simulink library "readers"  (R2020a)
settings: Solver=VariableStepAuto  StartTime=0.0  StopTime=10.0  RelTol=1e-3
settings Model: Creator=thomas  LastModifiedBy=thomas

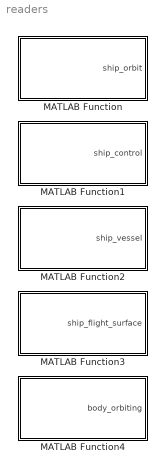
== system readers ==
  MATLAB Function : MATLAB Function  TreatAsAtomicUnit=on
  MATLAB Function1 : MATLAB Function  TreatAsAtomicUnit=on
  MATLAB Function2 : MATLAB Function  TreatAsAtomicUnit=on
  MATLAB Function3 : MATLAB Function  TreatAsAtomicUnit=on
  MATLAB Function4 : MATLAB Function  TreatAsAtomicUnit=on

== matlab function readers/MATLAB Function1 ==
  data: ship_control output Bus: ShipControl
function ship_control = read_control
    coder.extrinsic('evalin');
    ship_control.sas = false;
    ship_control.sas = evalin('base', 'vessel_control.getSAS();');
    ship_control.rcs = false;
    ship_control.rcs = evalin('base', 'vessel_control.getRCS();');
    ship_control.reaction_wheels = false;
    ship_control.reaction_wheels = evalin('base', 'vessel_control.getReactionWheels();');
    ship_control.gear = false;
    ship_control.gear = evalin('base', 'vessel_control.getGear();');
    ship_control.legs = false;
    ship_control.legs = evalin('base', 'vessel_control.getLegs();');
    ship_control.wheels = false;
    ship_control.wheels = evalin('base', 'vessel_control.getWheels();');
    ship_control.lights = false;
    ship_control.lights = evalin('base', 'vessel_control.getLights();');
    ship_control.brakes = false;
    ship_control.brakes = evalin('base', 'vessel_control.getBrakes();');
    ship_control.antennas = false;
    ship_control.antennas = evalin('base', 'vessel_control.getAntennas();');
    ship_control.cargo_bays = false;
    ship_control.cargo_bays = evalin('base', 'vessel_control.getCargoBays();');
    ship_control.intakes = false;
    ship_control.intakes = evalin('base', 'vessel_control.getIntakes();');
    ship_control.parachutes = false;
    ship_control.parachutes = evalin('base', 'vessel_control.getParachutes();');
    ship_control.radiators = false;
    ship_control.radiators = evalin('base', 'vessel_control.getRadiators();');
    ship_control.resource_harvesters = false;
    ship_control.resource_harvesters = evalin('base', 'vessel_control.getResourceHarvesters();');
    ship_control.resource_harvesters_active = false;
    ship_control.resource_harvesters_active = evalin('base', 'vessel_control.getResourceHarvestersActive();');
    ship_control.solar_panels = false;
    ship_control.solar_panels = evalin('base', 'vessel_control.getSolarPanels();');
    ship_control.abort = false;
    ship_control.abort = evalin('base', 'vessel_control.getAbort();');
    ship_control.throttle = 0.0;
    ship_control.throttle = evalin('base', 'vessel_control.getThrottle();');
    ship_control.pitch = 0.0;
    ship_control.pitch = evalin('base', 'vessel_control.getPitch();');
    ship_control.yaw = 0.0;
    ship_control.yaw = evalin('base', 'vessel_control.getYaw();');
    ship_control.roll = 0.0;
    ship_control.roll = evalin('base', 'vessel_control.getRoll();');
    ship_control.forward = 0.0;
    ship_control.forward = evalin('base', 'vessel_control.getForward();');
    ship_control.up = 0.0;
    ship_control.up = evalin('base', 'vessel_control.getUp();');
    ship_control.right = 0.0;
    ship_control.right = evalin('base', 'vessel_control.getRight();');
    ship_control.wheel_throttle = 0.0;
    ship_control.wheel_throttle = evalin('base', 'vessel_control.getWheelThrottle();');
    ship_control.wheel_steering = 0.0;
    ship_control.wheel_steering = evalin('base', 'vessel_control.getWheelSteering();');
    ship_control.current_stage = uint8(0);
    ship_control.current_stage = evalin('base', 'uint8(vessel_control.getCurrentStage());');
    
end

== matlab function readers/MATLAB Function ==
  data: ship_orbit output Bus: ShipOrbit
function ship_orbit = read_orbit
    coder.extrinsic('evalin');
    ship_orbit.apoapsis = 0.0;
    ship_orbit.apoapsis = evalin('base', 'vessel_orbit.getApoapsis();');
    ship_orbit.periapsis = 0.0;
    ship_orbit.periapsis = evalin('base', 'vessel_orbit.getPeriapsis();');
    ship_orbit.apoapsis_altitude = 0.0;
    ship_orbit.apoapsis_altitude = evalin('base', 'vessel_orbit.getApoapsisAltitude();');
    ship_orbit.periapsis_altitude = 0.0;
    ship_orbit.periapsis_altitude = evalin('base', 'vessel_orbit.getPeriapsisAltitude();');
    ship_orbit.semimajor_axis = 0.0;
    ship_orbit.semimajor_axis = evalin('base', 'vessel_orbit.getSemiMajorAxis();');
    ship_orbit.semiminor_axis = 0.0;
    ship_orbit.semiminor_axis = evalin('base', 'vessel_orbit.getSemiMinorAxis();');
    ship_orbit.radius = 0.0;
    ship_orbit.radius = evalin('base', 'vessel_orbit.getRadius();');
    ship_orbit.speed = 0.0;
    ship_orbit.speed = evalin('base', 'vessel_orbit.getSpeed();');
    ship_orbit.period = 0.0;
    ship_orbit.period = evalin('base', 'vessel_orbit.getPeriod();');
    ship_orbit.time_to_apoapsis = 0.0;
    ship_orbit.time_to_apoapsis = evalin('base', 'vessel_orbit.getTimeToApoapsis();');
    ship_orbit.time_to_periapsis = 0.0;
    ship_orbit.time_to_periapsis = evalin('base', 'vessel_orbit.getTimeToPeriapsis();');
    ship_orbit.eccentricity = 0.0;
    ship_orbit.eccentricity = evalin('base', 'vessel_orbit.getEccentricity();');
    ship_orbit.inclination = 0.0;
    ship_orbit.inclination = evalin('base', 'vessel_orbit.getInclination();');
    ship_orbit.longitude_of_ascending_node = 0.0;
    ship_orbit.longitude_of_ascending_node = evalin('base', 'vessel_orbit.getLongitudeOfAscendingNode();');
    ship_orbit.argument_of_periapsis = 0.0;
    ship_orbit.argument_of_periapsis = evalin('base', 'vessel_orbit.getArgumentOfPeriapsis();');
    ship_orbit.mean_anomaly_at_epoch = 0.0;
    ship_orbit.mean_anomaly_at_epoch = evalin('base', 'vessel_orbit.getMeanAnomalyAtEpoch();');
    ship_orbit.epoch = 0.0;
    ship_orbit.epoch = evalin('base', 'vessel_orbit.getEpoch();');
    ship_orbit.mean_anomaly = 0.0;
    ship_orbit.mean_anomaly = evalin('base', 'vessel_orbit.getMeanAnomaly();');
    ship_orbit.eccentric_anomaly = 0.0;
    ship_orbit.eccentric_anomaly = evalin('base', 'vessel_orbit.getEccentricAnomaly();');
    ship_orbit.true_anomaly = 0.0;
    ship_orbit.true_anomaly = evalin('base', 'vessel_orbit.getTrueAnomaly();');
    ship_orbit.orbital_speed = 0.0;
    ship_orbit.orbital_speed = evalin('base', 'vessel_orbit.getOrbitalSpeed();');
    ship_orbit.time_to_soi_change = 0.0;
    ship_orbit.time_to_soi_change = evalin('base', 'vessel_orbit.getTimeToSOIChange();');
end

== matlab function readers/MATLAB Function2 ==
  data: ship_vessel output Bus: ShipVessel
function ship_vessel = read_vessel
    coder.extrinsic('evalin');
    ship_vessel.recoverable = false;
    ship_vessel.recoverable = evalin('base', 'vessel.getRecoverable();');
    ship_vessel.met = 0.0;
    ship_vessel.met = evalin('base', 'vessel.getMET();');
    ship_vessel.crew_capacity = uint8(0);
    ship_vessel.crew_capacity = evalin('base', 'uint8(vessel.getCrewCapacity());');
    ship_vessel.crew_count = uint8(0);
    ship_vessel.crew_count = evalin('base', 'uint8(vessel.getCrewCount());');
    ship_vessel.mass = 0.0;
    ship_vessel.mass = evalin('base', 'vessel.getMass();');
    ship_vessel.dry_mass = 0.0;
    ship_vessel.dry_mass = evalin('base', 'vessel.getDryMass();');
    ship_vessel.thrust = 0.0;
    ship_vessel.thrust = evalin('base', 'vessel.getThrust();');
    ship_vessel.available_thrust = 0.0;
    ship_vessel.available_thrust = evalin('base', 'vessel.getAvailableThrust();');
    ship_vessel.max_thrust = 0.0;
    ship_vessel.max_thrust = evalin('base', 'vessel.getMaxThrust();');
    ship_vessel.max_vacuum_thrust = 0.0;
    ship_vessel.max_vacuum_thrust = evalin('base', 'vessel.getMaxVacuumThrust();');
    ship_vessel.specific_impulse = 0.0;
    ship_vessel.specific_impulse = evalin('base', 'vessel.getSpecificImpulse();');
    ship_vessel.vacuum_specific_impulse = 0.0;
    ship_vessel.vacuum_specific_impulse = evalin('base', 'vessel.getVacuumSpecificImpulse();');
    ship_vessel.kerbin_sea_level_specific_impulse = 0.0;
    ship_vessel.kerbin_sea_level_specific_impulse = evalin('base', 'vessel.getKerbinSeaLevelSpecificImpulse();');
    evalin('base', 'AAtmp_vessel = vessel.getMomentOfInertia();');
    ship_vessel.moment_of_inertia = zeros(1,3);
    ship_vessel.moment_of_inertia(1) = evalin('base', 'AAtmp_vessel.getValue(0);');
    ship_vessel.moment_of_inertia(2) = evalin('base', 'AAtmp_vessel.getValue(1);');
    ship_vessel.moment_of_inertia(3) = evalin('base', 'AAtmp_vessel.getValue(2);');
    evalin('base', 'AAtmp_vessel = vessel.getAvailableTorque();');
    ship_vessel.available_torque = zeros(2,3);
    ship_vessel.available_torque(1,1) = evalin('base', 'AAtmp_vessel.getValue(0).getValue(0);');
    ship_vessel.available_torque(1,2) = evalin('base', 'AAtmp_vessel.getValue(0).getValue(1);');
    ship_vessel.available_torque(1,3) = evalin('base', 'AAtmp_vessel.getValue(0).getValue(2);');
    ship_vessel.available_torque(2,1) = evalin('base', 'AAtmp_vessel.getValue(1).getValue(0);');
    ship_vessel.available_torque(2,2) = evalin('base', 'AAtmp_vessel.getValue(1).getValue(1);');
    ship_vessel.available_torque(2,3) = evalin('base', 'AAtmp_vessel.getValue(1).getValue(2);');
    evalin('base', 'AAtmp_vessel = vessel.position(vessel_regular_rf);');
    ship_vessel.position_reg = zeros(1,3);
    ship_vessel.position_reg(1) = evalin('base', 'AAtmp_vessel.getValue(0);');
    ship_vessel.position_reg(2) = evalin('base', 'AAtmp_vessel.getValue(1);');
    ship_vessel.position_reg(3) = evalin('base', 'AAtmp_vessel.getValue(2);');
    evalin('base', 'AAtmp_vessel = vessel.velocity(vessel_regular_rf);');
    ship_vessel.velocity_reg = zeros(1,3);
    ship_vessel.velocity_reg(1) = evalin('base', 'AAtmp_vessel.getValue(0);');
    ship_vessel.velocity_reg(2) = evalin('base', 'AAtmp_vessel.getValue(1);');
    ship_vessel.velocity_reg(3) = evalin('base', 'AAtmp_vessel.getValue(2);');
    evalin('base', 'AAtmp_vessel = vessel.rotation(vessel_regular_rf);');
    ship_vessel.rotation_reg = zeros(1,4);
    ship_vessel.rotation_reg(1) = evalin('base', 'AAtmp_vessel.getValue(3);');
    ship_vessel.rotation_reg(2) = evalin('base', 'AAtmp_vessel.getValue(0);');
    ship_vessel.rotation_reg(3) = evalin('base', 'AAtmp_vessel.getValue(1);');
    ship_vessel.rotation_reg(4) = evalin('base', 'AAtmp_vessel.getValue(2);');
    evalin('base', 'AAtmp_vessel = vessel.direction(vessel_regular_rf);');
    ship_vessel.direction_reg = zeros(1,3);
    ship_vessel.direction_reg(1) = evalin('base', 'AAtmp_vessel.getValue(0);');
    ship_vessel.direction_reg(2) = evalin('base', 'AAtmp_vessel.getValue(1);');
    ship_vessel.direction_reg(3) = evalin('base', 'AAtmp_vessel.getValue(2);');
    evalin('base', 'AAtmp_vessel = vessel.angularVelocity(vessel_regular_rf);');
    ship_vessel.angular_velocity_reg = zeros(3,1);
    ship_vessel.angular_velocity_reg(1) = evalin('base', 'AAtmp_vessel.getValue(0);');
    ship_vessel.angular_velocity_reg(2) = evalin('base', 'AAtmp_vessel.getValue(1);');
    ship_vessel.angular_velocity_reg(3) = evalin('base', 'AAtmp_vessel.getValue(2);');
    evalin('base', 'AAtmp_vessel = vessel.position(vessel_surface_rf);');
    ship_vessel.position_surface = zeros(1,3);
    ship_vessel.position_surface(1) = evalin('base', 'AAtmp_vessel.getValue(0);');
    ship_vessel.position_surface(2) = evalin('base', 'AAtmp_vessel.getValue(1);');
    ship_vessel.position_surface(3) = evalin('base', 'AAtmp_vessel.getValue(2);');
    evalin('base', 'AAtmp_vessel = vessel.velocity(vessel_surface_rf);');
    ship_vessel.velocity_surface = zeros(1,3);
    ship_vessel.velocity_surface(1) = evalin('base', 'AAtmp_vessel.getValue(0);');
    ship_vessel.velocity_surface(2) = evalin('base', 'AAtmp_vessel.getValue(1);');
    ship_vessel.velocity_surface(3) = evalin('base', 'AAtmp_vessel.getValue(2);');
    evalin('base', 'AAtmp_vessel = vessel.rotation(vessel_surface_rf);');
    ship_vessel.rotation_surface = zeros(1,4);
    ship_vessel.rotation_surface(1) = evalin('base', 'AAtmp_vessel.getValue(3);');
    ship_vessel.rotation_surface(2) = evalin('base', 'AAtmp_vessel.getValue(0);');
    ship_vessel.rotation_surface(3) = evalin('base', 'AAtmp_vessel.getValue(1);');
    ship_vessel.rotation_surface(4) = evalin('base', 'AAtmp_vessel.getValue(2);');
    evalin('base', 'AAtmp_vessel = vessel.direction(vessel_surface_rf);');
    ship_vessel.direction_surface = zeros(1,3);
    ship_vessel.direction_surface(1) = evalin('base', 'AAtmp_vessel.getValue(0);');
    ship_vessel.direction_surface(2) = evalin('base', 'AAtmp_vessel.getValue(1);');
    ship_vessel.direction_surface(3) = evalin('base', 'AAtmp_vessel.getValue(2);');
    evalin('base', 'AAtmp_avs = vessel.angularVelocity(vessel_surface_rf);');
    ship_vessel.angular_velocity_surface = zeros(3,1);
    ship_vessel.angular_velocity_surface(1) = evalin('base', 'AAtmp_avs.getValue(0);');
    ship_vessel.angular_velocity_surface(2) = evalin('base', 'AAtmp_avs.getValue(1);');
    ship_vessel.angular_velocity_surface(3) = evalin('base', 'AAtmp_avs.getValue(2);');
    evalin('base', 'AAtmp_vessel = vessel.position(vessel_orbital_rf);');
    ship_vessel.position_orbital = zeros(1,3);
    ship_vessel.position_orbital(1) = evalin('base', 'AAtmp_vessel.getValue(0);');
    ship_vessel.position_orbital(2) = evalin('base', 'AAtmp_vessel.getValue(1);');
    ship_vessel.position_orbital(3) = evalin('base', 'AAtmp_vessel.getValue(2);');
    evalin('base', 'AAtmp_vessel = vessel.velocity(vessel_orbital_rf);');
    ship_vessel.velocity_orbital = zeros(1,3);
    ship_vessel.velocity_orbital(1) = evalin('base', 'AAtmp_vessel.getValue(0);');
    ship_vessel.velocity_orbital(2) = evalin('base', 'AAtmp_vessel.getValue(1);');
    ship_vessel.velocity_orbital(3) = evalin('base', 'AAtmp_vessel.getValue(2);');
    evalin('base', 'AAtmp_vessel = vessel.rotation(vessel_orbital_rf);');
    ship_vessel.rotation_orbital = zeros(1,4);
    ship_vessel.rotation_orbital(1) = evalin('base', 'AAtmp_vessel.getValue(3);');
    ship_vessel.rotation_orbital(2) = evalin('base', 'AAtmp_vessel.getValue(0);');
    ship_vessel.rotation_orbital(3) = evalin('base', 'AAtmp_vessel.getValue(1);');
    ship_vessel.rotation_orbital(4) = evalin('base', 'AAtmp_vessel.getValue(2);');
    evalin('base', 'AAtmp_vessel = vessel.direction(vessel_orbital_rf);');
    ship_vessel.direction_orbital = zeros(1,3);
    ship_vessel.direction_orbital(1) = evalin('base', 'AAtmp_vessel.getValue(0);');
    ship_vessel.direction_orbital(2) = evalin('base', 'AAtmp_vessel.getValue(1);');
    ship_vessel.direction_orbital(3) = evalin('base', 'AAtmp_vessel.getValue(2);');
    evalin('base', 'AAtmp_vessel = vessel.angularVelocity(vessel_orbital_rf);');
    ship_vessel.angular_velocity_orbital = zeros(3,1);
    ship_vessel.angular_velocity_orbital(1) = evalin('base', 'AAtmp_vessel.getValue(0);');
    ship_vessel.angular_velocity_orbital(2) = evalin('base', 'AAtmp_vessel.getValue(1);');
    ship_vessel.angular_velocity_orbital(3) = evalin('base', 'AAtmp_vessel.getValue(2);');
end

== matlab function readers/MATLAB Function3 ==
  data: ship_flight_surface output Bus: ShipFlight
function ship_flight_surface = read_flight_surface
    coder.extrinsic('evalin');
    ship_flight_surface.gforce = 0.0;
    ship_flight_surface.gforce = evalin('base', 'vessel_flight.getGForce();');
    ship_flight_surface.mean_altitude = 0.0;
    ship_flight_surface.mean_altitude = evalin('base', 'vessel_flight.getMeanAltitude();');
    ship_flight_surface.surface_altitude = 0.0;
    ship_flight_surface.surface_altitude = evalin('base', 'vessel_flight.getSurfaceAltitude();');
    ship_flight_surface.bedrock_altitude = 0.0;
    ship_flight_surface.bedrock_altitude = evalin('base', 'vessel_flight.getBedrockAltitude();');
    ship_flight_surface.elevation = 0.0;
    ship_flight_surface.elevation = evalin('base', 'vessel_flight.getElevation();');
    ship_flight_surface.latitude = 0.0;
    ship_flight_surface.latitude = evalin('base', 'vessel_flight.getLatitude();');
    ship_flight_surface.longitude = 0.0;
    ship_flight_surface.longitude = evalin('base', 'vessel_flight.getLongitude();');
    evalin('base', 'AAtmp_fs = vessel_flight.getVelocity();');
    ship_flight_surface.velocity = zeros(1,3);
    ship_flight_surface.velocity(1) = evalin('base', 'AAtmp_fs.getValue(0);');
    ship_flight_surface.velocity(2) = evalin('base', 'AAtmp_fs.getValue(1);');
    ship_flight_surface.velocity(3) = evalin('base', 'AAtmp_fs.getValue(2);');
    ship_flight_surface.speed = 0.0;
    ship_flight_surface.speed = evalin('base', 'vessel_flight.getSpeed();');
    ship_flight_surface.horizontal_speed = 0.0;
    ship_flight_surface.horizontal_speed = evalin('base', 'vessel_flight.getHorizontalSpeed();');
    ship_flight_surface.vertical_speed = 0.0;
    ship_flight_surface.vertical_speed = evalin('base', 'vessel_flight.getVerticalSpeed();');
    evalin('base', 'AAtmp_fs = vessel_flight.getCenterOfMass();');
    ship_flight_surface.center_of_mass = zeros(1,3);
    ship_flight_surface.center_of_mass(1) = evalin('base', 'AAtmp_fs.getValue(0);');
    ship_flight_surface.center_of_mass(2) = evalin('base', 'AAtmp_fs.getValue(1);');
    ship_flight_surface.center_of_mass(3) = evalin('base', 'AAtmp_fs.getValue(2);');
    evalin('base', 'AAtmp_fs = vessel_flight.getRotation();');
    ship_flight_surface.rotation = zeros(1,4);
    ship_flight_surface.rotation(1) = evalin('base', 'AAtmp_fs.getValue(3);');
    ship_flight_surface.rotation(2) = evalin('base', 'AAtmp_fs.getValue(0);');
    ship_flight_surface.rotation(3) = evalin('base', 'AAtmp_fs.getValue(1);');
    ship_flight_surface.rotation(4) = evalin('base', 'AAtmp_fs.getValue(2);');
    evalin('base', 'AAtmp_fs = vessel_flight.getDirection();');
    ship_flight_surface.direction = zeros(1,3);
    ship_flight_surface.direction(1) = evalin('base', 'AAtmp_fs.getValue(0);');
    ship_flight_surface.direction(2) = evalin('base', 'AAtmp_fs.getValue(1);');
    ship_flight_surface.direction(3) = evalin('base', 'AAtmp_fs.getValue(2);');
    ship_flight_surface.pitch = 0.0;
    ship_flight_surface.pitch = evalin('base', 'vessel_flight.getPitch();');
    ship_flight_surface.heading = 0.0;
    ship_flight_surface.heading = evalin('base', 'vessel_flight.getHeading();');
    ship_flight_surface.roll = 0.0;
    ship_flight_surface.roll = evalin('base', 'vessel_flight.getRoll();');
    evalin('base', 'AAtmp_fs = vessel_flight.getPrograde();');
    ship_flight_surface.prograde = zeros(1,3);
    ship_flight_surface.prograde(1) = evalin('base', 'AAtmp_fs.getValue(0);');
    ship_flight_surface.prograde(2) = evalin('base', 'AAtmp_fs.getValue(1);');
    ship_flight_surface.prograde(3) = evalin('base', 'AAtmp_fs.getValue(2);');
    evalin('base', 'AAtmp_fs = vessel_flight.getRetrograde();');
    ship_flight_surface.retrograde = zeros(1,3);
    ship_flight_surface.retrograde(1) = evalin('base', 'AAtmp_fs.getValue(0);');
    ship_flight_surface.retrograde(2) = evalin('base', 'AAtmp_fs.getValue(1);');
    ship_flight_surface.retrograde(3) = evalin('base', 'AAtmp_fs.getValue(2);');
    evalin('base', 'AAtmp_fs = vessel_flight.getNormal();');
    ship_flight_surface.normal = zeros(1,3);
    ship_flight_surface.normal(1) = evalin('base', 'AAtmp_fs.getValue(0);');
    ship_flight_surface.normal(2) = evalin('base', 'AAtmp_fs.getValue(1);');
    ship_flight_surface.normal(3) = evalin('base', 'AAtmp_fs.getValue(2);');
    evalin('base', 'AAtmp_fs = vessel_flight.getAntiNormal();');
    ship_flight_surface.antinormal = zeros(1,3);
    ship_flight_surface.antinormal(1) = evalin('base', 'AAtmp_fs.getValue(0);');
    ship_flight_surface.antinormal(2) = evalin('base', 'AAtmp_fs.getValue(1);');
    ship_flight_surface.antinormal(3) = evalin('base', 'AAtmp_fs.getValue(2);');
    evalin('base', 'AAtmp_fs = vessel_flight.getRadial();');
    ship_flight_surface.radial = zeros(1,3);
    ship_flight_surface.radial(1) = evalin('base', 'AAtmp_fs.getValue(0);');
    ship_flight_surface.radial(2) = evalin('base', 'AAtmp_fs.getValue(1);');
    ship_flight_surface.radial(3) = evalin('base', 'AAtmp_fs.getValue(2);');
    evalin('base', 'AAtmp_fs = vessel_flight.getAntiRadial();');
    ship_flight_surface.antiradial = zeros(1,3);
    ship_flight_surface.antiradial(1) = evalin('base', 'AAtmp_fs.getValue(0);');
    ship_flight_surface.antiradial(2) = evalin('base', 'AAtmp_fs.getValue(1);');
    ship_flight_surface.antiradial(3) = evalin('base', 'AAtmp_fs.getValue(2);');
    ship_flight_surface.atmosphere_density = 0.0;
    ship_flight_surface.atmosphere_density = evalin('base', 'vessel_flight.getAtmosphereDensity();');
    ship_flight_surface.dynamic_pressure = 0.0;
    ship_flight_surface.dynamic_pressure = evalin('base', 'vessel_flight.getDynamicPressure();');
    ship_flight_surface.static_pressure = 0.0;
    ship_flight_surface.static_pressure = evalin('base', 'vessel_flight.getStaticPressure();');
    ship_flight_surface.static_pressure_at_msl = 0.0;
    ship_flight_surface.static_pressure_at_msl = evalin('base', 'vessel_flight.getStaticPressureAtMSL();');
    evalin('base', 'AAtmp_fs = vessel_flight.getAerodynamicForce();');
    ship_flight_surface.aerodynamic_force = zeros(1,3);
    ship_flight_surface.aerodynamic_force(1) = evalin('base', 'AAtmp_fs.getValue(0);');
    ship_flight_surface.aerodynamic_force(2) = evalin('base', 'AAtmp_fs.getValue(1);');
    ship_flight_surface.aerodynamic_force(3) = evalin('base', 'AAtmp_fs.getValue(2);');
    evalin('base', 'AAtmp_fs = vessel_flight.getLift();');
    ship_flight_surface.lift = zeros(1,3);
    ship_flight_surface.lift(1) = evalin('base', 'AAtmp_fs.getValue(0);');
    ship_flight_surface.lift(2) = evalin('base', 'AAtmp_fs.getValue(1);');
    ship_flight_surface.lift(3) = evalin('base', 'AAtmp_fs.getValue(2);');
    evalin('base', 'AAtmp_fs = vessel_flight.getDrag();');
    ship_flight_surface.drag = zeros(1,3);
    ship_flight_surface.drag(1) = evalin('base', 'AAtmp_fs.getValue(0);');
    ship_flight_surface.drag(2) = evalin('base', 'AAtmp_fs.getValue(1);');
    ship_flight_surface.drag(3) = evalin('base', 'AAtmp_fs.getValue(2);');
    ship_flight_surface.speed_of_sound = 0.0;
    ship_flight_surface.speed_of_sound = evalin('base', 'vessel_flight.getSpeedOfSound();');
    ship_flight_surface.mach = 0.0;
    ship_flight_surface.mach = evalin('base', 'vessel_flight.getMach();');
    ship_flight_surface.true_air_speed = 0.0;
    ship_flight_surface.true_air_speed = evalin('base', 'vessel_flight.getTrueAirSpeed();');
    ship_flight_surface.equivalent_air_speed = 0.0;
    ship_flight_surface.equivalent_air_speed = evalin('base', 'vessel_flight.getEquivalentAirSpeed();');
    ship_flight_surface.terminal_velocity = 0.0;
    ship_flight_surface.terminal_velocity = evalin('base', 'vessel_flight.getTerminalVelocity();');
    ship_flight_surface.angle_of_attack = 0.0;
    ship_flight_surface.angle_of_attack = evalin('base', 'vessel_flight.getAngleOfAttack();');
    ship_flight_surface.sideslip_angle = 0.0;
    ship_flight_surface.sideslip_angle = evalin('base', 'vessel_flight.getSideslipAngle();');
    ship_flight_surface.total_air_temperature = 0.0;
    ship_flight_surface.total_air_temperature = evalin('base', 'vessel_flight.getTotalAirTemperature();');
    ship_flight_surface.static_air_temperature = 0.0;
    ship_flight_surface.static_air_temperature = evalin('base', 'vessel_flight.getStaticAirTemperature();');

end

== matlab function readers/MATLAB Function4 ==
  data: body_orbiting output Bus: CelestialBody
function body_orbiting = read_body_orbiting
    coder.extrinsic('evalin');
    body_orbiting.mass = 0.0;
    body_orbiting.mass = evalin('base', 'vessel_orbit.getBody().getMass();');
    body_orbiting.gravitational_parameter = 0.0;
    body_orbiting.gravitational_parameter = evalin('base', 'vessel_orbit.getBody().getGravitationalParameter();');
    body_orbiting.surface_gravity = 0.0;
    body_orbiting.surface_gravity = evalin('base', 'vessel_orbit.getBody().getSurfaceGravity();');
    body_orbiting.rotational_period = 0.0;
    body_orbiting.rotational_period = evalin('base', 'vessel_orbit.getBody().getRotationalPeriod();');
    body_orbiting.rotational_speed = 0.0;
    body_orbiting.rotational_speed = evalin('base', 'vessel_orbit.getBody().getRotationalSpeed();');
    body_orbiting.rotation_angle = 0.0;
    body_orbiting.rotation_angle = evalin('base', 'vessel_orbit.getBody().getRotationAngle();');
    body_orbiting.initial_rotation = 0.0;
    body_orbiting.initial_rotation = evalin('base', 'vessel_orbit.getBody().getInitialRotation();');
    body_orbiting.equatorial_radius = 0.0;
    body_orbiting.equatorial_radius = evalin('base', 'vessel_orbit.getBody().getEquatorialRadius();');
    body_orbiting.sphere_of_influence = 0.0;
    body_orbiting.sphere_of_influence = evalin('base', 'vessel_orbit.getBody().getSphereOfInfluence();');
    body_orbiting.has_atmosphere = false;
    body_orbiting.has_atmosphere = evalin('base', 'vessel_orbit.getBody().getHasAtmosphere();');
    body_orbiting.atmosphere_depth = 0.0;
    body_orbiting.atmosphere_depth = evalin('base', 'vessel_orbit.getBody().getAtmosphereDepth();');
    body_orbiting.has_atmospheric_oxygen = false;
    body_orbiting.has_atmospheric_oxygen = evalin('base', 'vessel_orbit.getBody().getHasAtmosphericOxygen();');
    
end
